simulink model "realtime44"  (R2024b)
settings: Solver=ode5  StartTime=0.0  StopTime=4  FixedStep=0.001  RelTol=1e-3
undefined symbols (not defined in the file): degs2rpm, feedback, filt, National_Instruments, PCIe, rpm2rads, sens
libraries: sldrtlib x3, simulink x1
settings Model: SimulationMode=external  ExtModeTrigDuration=4001  Creator=ControlSystemsUser  LastModifiedBy=ControlSystemsUser
settings DataIOCC: ReturnWorkspaceOutputs=off
settings HardwareCC: ProdBitPerLong=64  ProdHWDeviceType=Intel->x86-64 (Linux 64)
settings RTWCC: Description=Simulink Desktop Real-Time  SystemTargetFile=sldrt.tlc  TemplateMakefile=sldrt.tmf  RTWCompilerOptimization=on
settings CodeAppCC: MaxIdLength=95
settings SimulinkDesktopRealTimeCC: TargetLibSuffix=_sldrt.a  TargetPreCompLibLocation=C:\Program Files\MATLAB\R2024b\toolbox\sldrt\lib\win64  ParMdlRefBuildCompliant=on

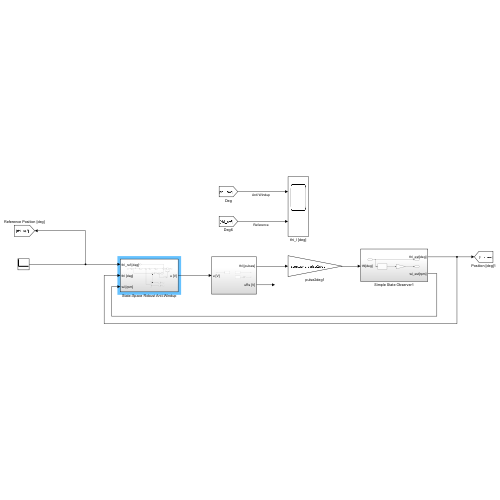
[thumbnail: Simulink's stored preview of the top-level diagram]
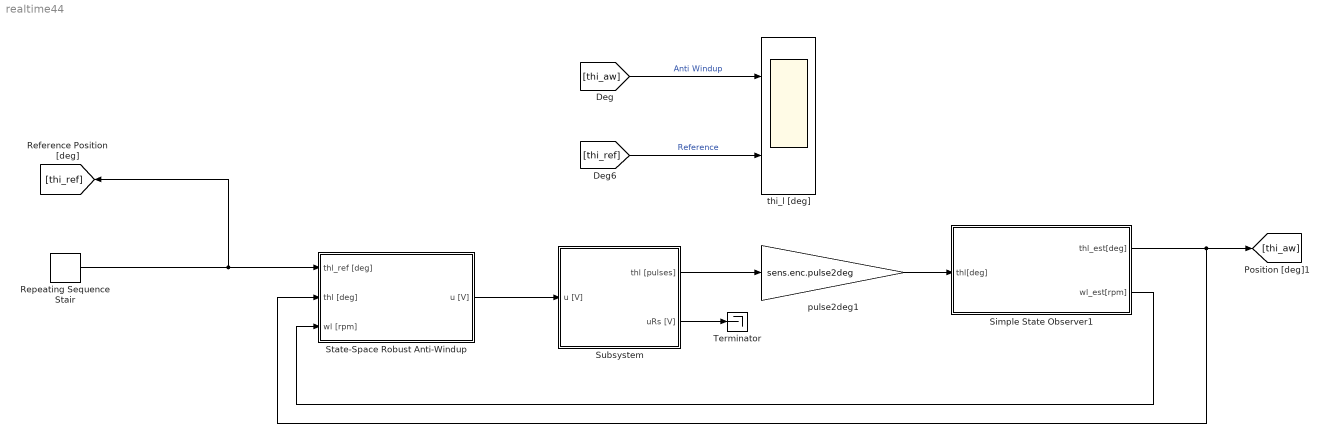
== system realtime44 ==
  Repeating Sequence Stair : simulink/Sources/Repeating Sequence Stair  OutValues=sIn.position  tsamp=sIn.sample_time  OutMin=[]  OutMax=[]  OutDataTypeStr=double  OutputDataTypeScalingMode=double  OutDataType=fixdt(0,8)  ConRadixGroup=Best Precision: Vector-wise  OutScaling=2^-12
  Simple State Observer1 : Subsystem
  State-Space Robust Anti-Windup : Subsystem
  Subsystem : Subsystem
  Terminator : Terminator
  pulse2deg1 : Gain  Gain=sens.enc.pulse2deg
  thi_l [deg] : Scope  NumInputPorts=2
  wires:
  Repeating Sequence Stair/1 -> [thi_ref], State-Space Robust Anti-Windup/1(thl_ref [deg])
  [thi_aw] -> thi_l [deg]/1  "Anti Windup"
  Subsystem/1(thl [pulses]) -> pulse2deg1/1
  State-Space Robust Anti-Windup/1(u [V]) -> Subsystem/1(u [V])
  [thi_ref] -> thi_l [deg]/2  "Reference"
  Simple State Observer1/2(wl_est[rpm]) -> State-Space Robust Anti-Windup/3(wl [rpm])
  Subsystem/2(uRs [V]) -> Terminator/1
  Simple State Observer1/1(thl_est[deg]) -> State-Space Robust Anti-Windup/2(thl [deg]), [thi_aw]
  pulse2deg1/1 -> Simple State Observer1/1(thl[deg])

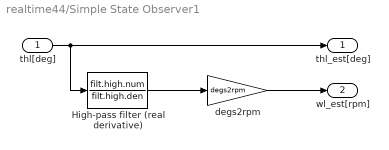
== system realtime44/Simple State Observer1 ==
  thl[deg] : Inport
  High-pass filter (real derivative) : TransferFcn  Numerator=filt.high.num  Denominator=filt.high.den
  degs2rpm : Gain  Gain=degs2rpm
  thl_est[deg] : Outport
  wl_est[rpm] : Outport  Port=2
  wires:
  thl[deg]/1 -> High-pass filter (real derivative)/1, thl_est[deg]/1
  High-pass filter (real derivative)/1 -> degs2rpm/1
  degs2rpm/1 -> wl_est[rpm]/1

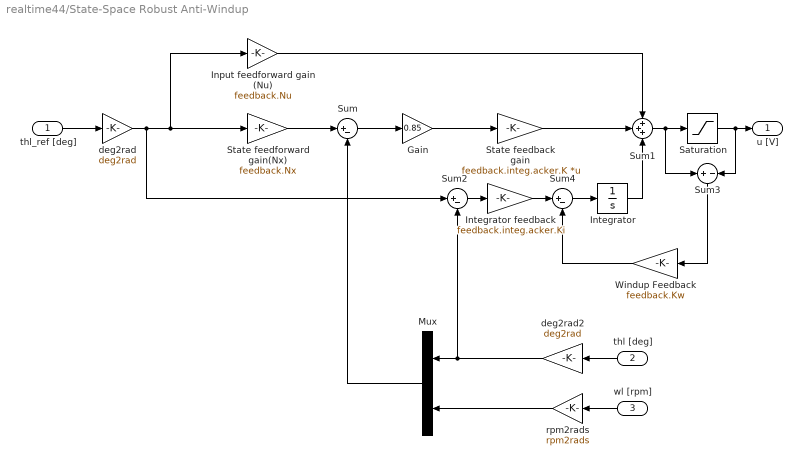
== system realtime44/State-Space Robust Anti-Windup ==
  thl_ref [deg] : Inport
  thl [deg] : Inport  Port=2
  wl [rpm] : Inport  Port=3
  Gain : Gain  Gain=0.85
  Input feedforward gain (Nu) : Gain  Gain=feedback.Nu
  Integrator : Integrator
  Integrator feedback : Gain  Gain=feedback.integ.acker.Ki
  Mux : Mux  Inputs=2
  Saturation : Saturate  UpperLimit=10  LowerLimit=-10
  State feedback gain : Gain  Gain=feedback.integ.acker.K  Multiplication=Matrix(K*u)
  State feedforward gain(Nx) : Gain  Gain=feedback.Nx
  Sum : Sum  Inputs=|+-
  Sum1 : Sum  Inputs=+++
  Sum2 : Sum  Inputs=|+-
  Sum3 : Sum  Inputs=+|-
  Sum4 : Sum  Inputs=|+-
  Windup Feedback : Gain  Gain=feedback.Kw
  deg2rad : Gain  Gain=deg2rad
  deg2rad2 : Gain  Gain=deg2rad
  rpm2rads : Gain  Gain=rpm2rads
  u [V] : Outport
  wires:
  thl_ref [deg]/1 -> deg2rad/1
  deg2rad/1 -> Sum2/1, Input feedforward gain (Nu)/1, State feedforward gain(Nx)/1
  State feedforward gain(Nx)/1 -> Sum/1
  Sum/1 -> Gain/1
  State feedback gain/1 -> Sum1/2
  Input feedforward gain (Nu)/1 -> Sum1/1
  Sum1/1 -> Saturation/1, Sum3/1
  Saturation/1 -> Sum3/2, u [V]/1
  thl [deg]/1 -> deg2rad2/1
  wl [rpm]/1 -> rpm2rads/1
  deg2rad2/1 -> Mux/1, Sum2/2
  rpm2rads/1 -> Mux/2
  Mux/1 -> Sum/2
  Sum2/1 -> Integrator feedback/1
  Integrator/1 -> Sum1/3
  Sum3/1 -> Windup Feedback/1
  Integrator feedback/1 -> Sum4/1
  Sum4/1 -> Integrator/1
  Windup Feedback/1 -> Sum4/2
  Gain/1 -> State feedback gain/1

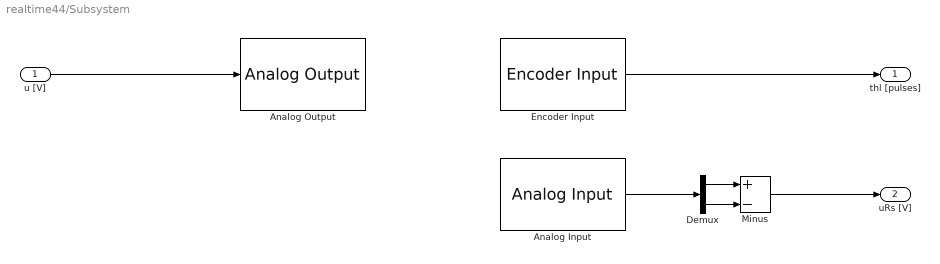
== system realtime44/Subsystem ==
  u [V] : Inport
  Analog Input : sldrtlib/Analog Input  SampleTime=-1  MaxMissedTicks=10  ShowMissedTicks=off  YieldWhenWaiting=off  DrvName=National_Instruments/PCIe-6321  DrvAddress=4294967295  DrvOptions=[0 0 0 2 0 0 0]  Channels=[1,2]  RangeMode=1  VoltRange=1  DataType=1
      settings: AttributesFormatString=National Instruments\nPCIe-6321 [auto]
  Analog Output : sldrtlib/Analog Output  SampleTime=-1  MaxMissedTicks=10  ShowMissedTicks=off  YieldWhenWaiting=off  DrvName=National_Instruments/PCIe-6321  DrvAddress=4294967295  DrvOptions=[0 0 0 2 0 0 0]  Channels=1  RangeMode=1  VoltRange=1  InitialValue=0  FinalValue=0
      settings: AttributesFormatString=National Instruments\nPCIe-6321 [auto]
  Demux : Demux  Outputs=2
  Encoder Input : sldrtlib/Encoder Input  SampleTime=-1  MaxMissedTicks=10  ShowMissedTicks=off  YieldWhenWaiting=off  DrvName=National_Instruments/PCIe-6321  DrvAddress=4294967295  DrvOptions=[0 0 0 2 0 0 0]  Channels=1  QuadMode=3  IndexPulse=1  InputFilter=Inf  DataType=1
      settings: AttributesFormatString=National Instruments\nPCIe-6321 [auto]
  Minus : Sum  Inputs=+-
  thl [pulses] : Outport
  uRs [V] : Outport  Port=2
  wires:
  Minus/1 -> uRs [V]/1
  Analog Input/1 -> Demux/1
  Demux/1 -> Minus/1
  Demux/2 -> Minus/2
  Encoder Input/1 -> thl [pulses]/1
  u [V]/1 -> Analog Output/1
